simulink model "simLQR"  (R2022b)
settings: Solver=ode45  StartTime=0.0  StopTime=inf  RelTol=1e-3
undefined symbols (not defined in the file or in its folder): Angular, curvature, DiscIntNeverNeededParam, esc, hz, Linear, path, Q, R_, velocity
libraries: robotlib x4, dspstat3 x1
settings Model: Creator=kisho  LastModifiedBy=kishor
settings OptimizationCC: DefaultParameterBehavior=Inlined  EnhancedBackFolding=on  PassReuseOutputArgsAs=Individual arguments  ZeroExternalMemoryAtStartup=off  ZeroInternalMemoryAtStartup=off  MaxStackSize=64  OptimizeBlockOrder=speed  DifferentSizesBufferReuse=on  OptimizationCustomize=off  EfficientTunableParamExpr=on
settings DebuggingCC: ParameterTunabilityLossMsg=error  UnconnectedInputMsg=warning  UnconnectedOutputMsg=warning  UnconnectedLineMsg=warning
settings HardwareCC: ProdBitPerPointer=32  ProdBitPerSizeT=32  ProdBitPerPtrDiffT=32  ProdLargestAtomicFloat=None  ProdIntDivRoundTo=Undefined  ProdEndianess=Unspecified  ProdWordSize=32  ProdHWDeviceType=ASIC/FPGA->ASIC/FPGA  TargetBitPerLong=64  TargetBitPerPointer=64  TargetBitPerSizeT=64  TargetBitPerPtrDiffT=64  TargetLongLongMode=on  TargetIntDivRoundTo=Zero  TargetEndianess=LittleEndian  TargetWordSize=64  TargetHWDeviceType=Custom Processor->MATLAB Host Computer  ProdEqTarget=off
settings ModelReferenceCC: EnableRefExpFcnMdlSchedulingChecks=on
settings SFSimCC: MATLABDynamicMemAlloc=off
settings RTWCC: Description=Embedded Coder  SystemTargetFile=ert.tlc  TemplateMakefile=ert_default_tmf  Toolchain=Catkin  DLArmComputeVersion=19.05
settings CodeAppCC: ForceParamTrailComments=on  IgnoreCustomStorageClasses=off  OperatorAnnotations=on  SimulinkDataObjDesc=on  SFDataObjDesc=on  InsertBlockDesc=on
settings ERTTargetCC: InlinedParameterPlacement=NonHierarchical  ERTCustomFileTemplate=example_file_process.tlc

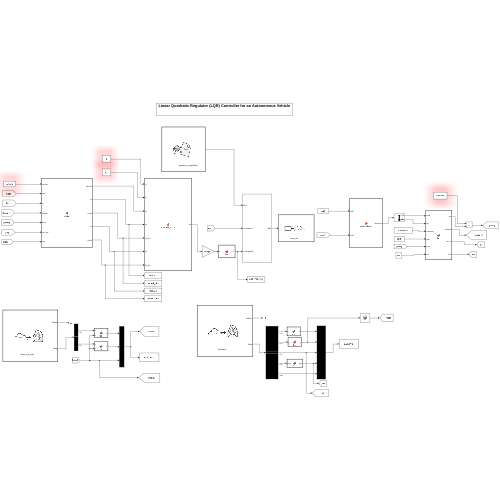
[thumbnail: Simulink's stored preview of the top-level diagram]
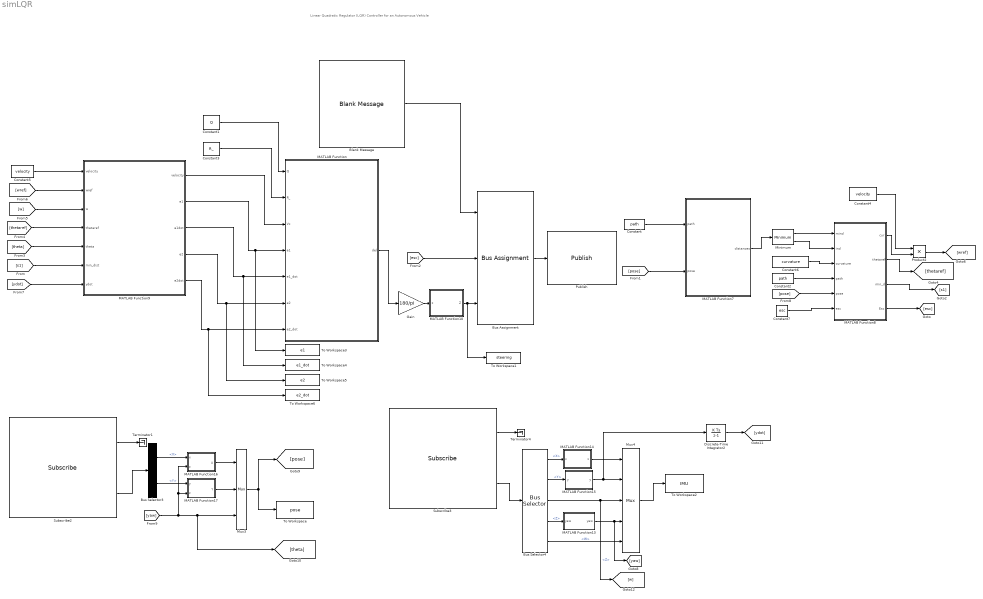
== system simLQR ==
  note: Linear Quadratic Regulator (LQR) Controller for an Autonomous Vehicle
  Blank Message : robotlib/Blank Message  messageClass=Message  entityType=geometry_msgs/Twist  messageType=geometry_msgs/Twist  SampleTime=1/hz  legacyBusStruct=off
      settings: LibrarySourceBlock=roslib/ROS/Blank Message
  Bus Assignment : BusAssignment  AssignedSignals=Linear.X,Angular.Z
  Bus Selector3 : BusSelector  OutputSignals=Pose.Position.X,Pose.Position.Y
  Bus Selector4 : BusSelector  OutputSignals=LinearAcceleration.X,LinearAcceleration.Y,AngularVelocity.Z,Orientation.Z,Orientation.W
  Constant : Constant  Value=path  SampleTime=1/hz
  Constant1 : Constant  Value=Q  SampleTime=1/hz
  Constant2 : Constant  Value=path  SampleTime=1/hz
  Constant3 : Constant  Value=R_  SampleTime=1/hz
  Constant4 : Constant  Value=velocity  SampleTime=1/hz
  Constant5 : Constant  Value=velocity  SampleTime=1/hz
  Constant6 : Constant  Value=curvature  SampleTime=1/hz
  Constant7 : Constant  Value=esc  SampleTime=1/hz
  Discrete-Time Integrator2 : DiscreteIntegrator  SampleTime=1/hz  ICPrevOutput=DiscIntNeverNeededParam  ICPrevScaledInput=DiscIntNeverNeededParam
  Gain : Gain  Gain=180/pi
  MATLAB Function : MATLAB Function  TreatAsAtomicUnit=on
  MATLAB Function10 : MATLAB Function  TreatAsAtomicUnit=on
  MATLAB Function13 : MATLAB Function  TreatAsAtomicUnit=on
  MATLAB Function14 : MATLAB Function  TreatAsAtomicUnit=on
  MATLAB Function15 : MATLAB Function  TreatAsAtomicUnit=on
  MATLAB Function16 : MATLAB Function  TreatAsAtomicUnit=on
  MATLAB Function17 : MATLAB Function  TreatAsAtomicUnit=on
  MATLAB Function7 : MATLAB Function  TreatAsAtomicUnit=on
  MATLAB Function8 : MATLAB Function  TreatAsAtomicUnit=on
  MATLAB Function9 : MATLAB Function  TreatAsAtomicUnit=on
  Minimum : dspstat3/Minimum  operation=minimum  fcn=Value and Index  indexBase=One  operateOver=Each row  Dimension=1  InputProcessing=Columns as channels (frame based)  reset=None  roiEnable=off  roiType=Rectangles  roiPortion=Entire ROI  roiOutput=Individual statistics for each ROI  roiFlag=off  roundingMode=Floor  overflowMode=off
  Mux3 : Mux  Inputs=3
  Mux4 : Mux  Inputs=5
  Product2 : Product
  Publish : robotlib/Publish  topicSource=Specify your own  topic=/cmd_vel  messageType=geometry_msgs/Twist  legacyBusStruct=off  messageQueueLength=1
      settings: LibrarySourceBlock=roslib/ROS/Publish
  Subscribe2 : robotlib/Subscribe  topicSource=Specify your own  topic=/slam_out_pose  messageType=geometry_msgs/PoseStamped  SampleTime=1/hz  legacyBusStruct=off  messageQueueLength=1
      settings: LibrarySourceBlock=roslib/ROS/Subscribe
  Subscribe3 : robotlib/Subscribe  topicSource=Specify your own  topic=/imu/data  messageType=sensor_msgs/Imu  SampleTime=1/hz  legacyBusStruct=off  messageQueueLength=1
      settings: LibrarySourceBlock=roslib/ROS/Subscribe
  Terminator1 : Terminator
  Terminator4 : Terminator
  To Workspace : ToWorkspace  VariableName=pose  SaveFormat=Structure With Time  SampleTime=-1
  To Workspace1 : ToWorkspace  VariableName=steering  SaveFormat=Structure With Time  SampleTime=-1
  To Workspace2 : ToWorkspace  VariableName=IMU  SaveFormat=Structure With Time  SampleTime=-1
  To Workspace3 : ToWorkspace  VariableName=e1  SaveFormat=Structure With Time  SampleTime=-1
  To Workspace4 : ToWorkspace  VariableName=e1_dot  SaveFormat=Structure With Time  SampleTime=-1
  To Workspace5 : ToWorkspace  VariableName=e2  SaveFormat=Structure With Time  SampleTime=-1
  To Workspace6 : ToWorkspace  VariableName=e2_dot  SaveFormat=Structure With Time  SampleTime=-1
  wires:
  MATLAB Function/1(del) -> Gain/1
  Bus Assignment/1 -> Publish/1
  Blank Message/1 -> Bus Assignment/1
  Gain/1 -> MATLAB Function10/1(z)
  [s1] -> MATLAB Function9/6(min_dist)
  [theta] -> MATLAB Function9/5(theta)
  [thetaref] -> MATLAB Function9/4(thetaref)
  [w] -> MATLAB Function9/3(w)
  [wref] -> MATLAB Function9/2(wref)
  Constant5/1 -> MATLAB Function9/1("velocity ")
  [ydot] -> MATLAB Function9/7(ydot)
  MATLAB Function9/2(e1) -> To Workspace3/1, MATLAB Function/4(e1)
  MATLAB Function9/3(e1dot) -> To Workspace4/1, MATLAB Function/5(e1_dot)
  MATLAB Function9/4(e2) -> To Workspace5/1, MATLAB Function/6(e2)
  MATLAB Function9/5(e2dot) -> To Workspace6/1, MATLAB Function/7(e2_dot)
  MATLAB Function9/1(velocity) -> MATLAB Function/3(Vx)
  Constant3/1 -> MATLAB Function/2(R_)
  Constant1/1 -> MATLAB Function/1(Q)
  [esc] -> Bus Assignment/2
  Minimum/2 -> MATLAB Function8/2(ind)
  Constant/1 -> MATLAB Function7/1(path)
  MATLAB Function8/3(min_d) -> [s1]
  MATLAB Function8/4(Esc) -> [esc]
  [pose] -> MATLAB Function8/5(pose)
  [pose] -> MATLAB Function7/2(pose)
  Constant4/1 -> Product2/1
  Product2/1 -> [wref]
  MATLAB Function8/1(cur) -> Product2/2
  MATLAB Function7/1(distances) -> Minimum/1
  Constant6/1 -> MATLAB Function8/3(curvature)
  MATLAB Function8/2(thetaref) -> [thetaref]
  Constant7/1 -> MATLAB Function8/6(esc)
  Minimum/1 -> MATLAB Function8/1(mind)
  Constant2/1 -> MATLAB Function8/4(path)
  [yaw] -> [theta], Mux3/3, MATLAB Function16/2(z), MATLAB Function17/2(z)
  MATLAB Function16/1(X) -> Mux3/1
  Bus Selector4/2 -> MATLAB Function15/1("y ")  "<Y>"
  MATLAB Function13/1(yaw) -> [yaw], Mux4/4
  Mux3/1 -> [pose], To Workspace/1
  MATLAB Function15/1(y) -> Discrete-Time Integrator2/1, Mux4/2
  Subscribe2/2 -> Bus Selector3/1
  Bus Selector4/1 -> MATLAB Function14/1("x ")  "<X>"
  Subscribe3/2 -> Bus Selector4/1
  Mux4/1 -> To Workspace2/1
  Bus Selector4/4 -> MATLAB Function13/1("yaw ")  "<Z>"
  Subscribe3/1 -> Terminator4/1
  Subscribe2/1 -> Terminator1/1
  MATLAB Function14/1(x) -> Mux4/1
  Bus Selector3/2 -> MATLAB Function17/1(y)  "<Y>"
  MATLAB Function17/1(Y) -> Mux3/2
  Bus Selector3/1 -> MATLAB Function16/1(x)  "<X>"
  Discrete-Time Integrator2/1 -> [ydot]
  Bus Selector4/3 -> [w], Mux4/3  "<Z>"
  Bus Selector4/5 -> Mux4/5  "<W>"
  MATLAB Function10/1(Z) -> To Workspace1/1, Bus Assignment/3

== matlab function simLQR/MATLAB Function17 ==
  data: y input; Y output; z input
function Y = fcn(y,z)
Y = y + 0.330*sin(z)/2;
end

== matlab function simLQR/MATLAB Function ==
  data: Q input; R_ input; del output; Vx input; e1 input; e1_dot input; e2 input; e2_dot input
function del = steering_angle(Q,R_,Vx,e1,e1_dot, e2, e2_dot)

% defining vehicle parameters
a = 0.330/2;     % m ,distance from CoG to front axel
b = 0.330/2;     % m ,distance from CoG to rear axel
Iz = 5*0.1^2;  % kg-m^2 ,Yaw rate of inertia around CoG
m = 5;     % kg ,mass of the vehicle 
Cf = 8354;   % N/rad ,cornering stiffness of the front axel
Cr = 8310;   % N/rad ,cornering stiffness of the rear axel
w = 0.25 ;   % m ,vehicle width
lf = 0.330/2;    % m ,CoG to front end 
lr = 0.330/2;    % m ,CoG to rear end

% state space and control inpute's coefficient matrix
A = [0,1,0,0;
    0,-(2*Cf+2*Cr)/(m*Vx),(2*Cf+2*Cf)/(m),(-2*Cf*lf+2*Cf*lr)/(m*Vx);
    0,0,0,1;
    0,-(2*Cf*lf-2*Cf*lr)/(Iz*Vx),(2*Cf*lf-2*Cf*lr)/(Iz),-(2*Cf*lf^2+2*Cf*lr^2)/(Iz*Vx)];

B1 = [0; ((-2*Cf+Cf)/(m*Vx)-Vx); 0; -(2*Cf*lf^2+2*Cf*lr^2)/(Iz*Vx)];

B = [0; (2*Cf/m); 0; (2*Cf*lf/Iz)];

B2 = [0;0;0;1];
%Q = diag([5 0 5 1]);
%R = 10;

% calculating gain matrix
K = lqr_own(A, B, Q, R_);

% state space matrix
X = [e1;e1_dot; e2; e2_dot];



del = [-K*X];

== matlab function simLQR/MATLAB Function7 ==
  data: path input; distances output; pose input
function distances  = nearestPose(path, pose)
    % path: Nx3 matrix containing the x, y, and heading of the waypoints in the path
    % current_pose: 1x3 vector containing the x, y, and heading of the current pose of the vehicle
    % nearest_pose: 1x3 vector containing the x, y, and heading of the nearest pose on the path
    % nearest_index: index of the nearest pose on the path
    
    % Find the distance from the current pose to each waypoint on the path
    
    l = length(path(:,1));
    cx = path(:,1);
    cy = path(:,2);
    dx = zeros(l);
    dy = zeros(l);
    distances =  zeros(1,l);


    for i = 1:l
        dx(i) = pose(1) - cx(i);
        dy(i) = pose(2) - cy(i);
        distances(i) = sqrt((dx(i)^2+dy(i)^2));
    end
end

== matlab function simLQR/MATLAB Function8 ==
  data: mind input; ind input; curvature input; cur output; path input; thetaref output; pose input; min_d output; esc input; Esc output
function [cur,thetaref,min_d,Esc] = fcn(mind,ind,curvature,path,pose,esc)

cur = curvature(ind);
thetaref = path(ind,3);

% cross track error

current_position = [pose(1);pose(2)];
next_waypoint = [path(ind+1,1);path(ind+1,2)];

waypoint_vector = next_waypoint - current_position;
normal_vector = [-waypoint_vector(2), waypoint_vector(1)];
vehicle_heading = [cos(pose(3)), sin(pose(3))];
dot_product = dot(vehicle_heading, normal_vector);
if dot_product > 0
    cross_track_error = +1; % vehicle is to the right of the line
else
    cross_track_error = -1; % vehicle is to the left of the line
end
min_d = mind*cross_track_error;


%%% stopping the vehicle when vehicle reaching near the target point

if (ind >= length(path)-20)
    Esc = 0;
else
    Esc = esc;
end

end

== matlab function simLQR/MATLAB Function9 ==
  data: velocity output; velocity input; wref input; e1 output; e1dot output; e2 output; e2dot output; w input; thetaref input; theta input; min_dist input; ydot input
function [velocity,e1,e1dot,e2,e2dot]= state(velocity,wref,w,thetaref,theta,min_dist,ydot)

% rate change of heading error
 e2dot = w - wref;

% heading error 
 e2    = theta -thetaref;
if e2 <= -pi
    e2 = theta + (2*pi-thetaref);
elseif e2 >= pi
    e2 = -(2*pi-theta+thetaref);
end
a = e2*180/pi
% cross track error
 e1 = min_dist;
 e1dot = ydot+velocity*(e2);
end

== matlab function simLQR/MATLAB Function10 ==
  data: z input; Z output
function Z = fcn(z)

if (z > 30)
    z = 30;
elseif (z < -30)
    z = -30;
else
    z =z;
end

Z = z;
end

== matlab function simLQR/MATLAB Function13 ==
  data: yaw input; yaw output
function yaw = fcn(yaw)
yaw = 360-yaw;

yaw = yaw*pi/180;
end

== matlab function simLQR/MATLAB Function14 ==
  data: x input; x output
function x = fcn(x)
x = x - (0);
end

== matlab function simLQR/MATLAB Function15 ==
  data: y input; y output
function y = fcn(y)
y = y - (0);
end

== matlab function simLQR/MATLAB Function16 ==
  data: x input; X output; z input
function X = fcn(x,z)

X = x + 0.330*cos(z)/2;

end
